simulink model "faults"  (R2023b)
settings: Solver=VariableStepAuto  StartTime=0.0  StopTime=10.0  RelTol=1e-3
libraries: spsSeriesRLCBranchLib x4, spsThreePhaseBreakerLib x1, spsThreePhaseFaultLib x1, spsUniversalBridgeLib x1
settings Model: Creator=edemk  LastModifiedBy=edemk

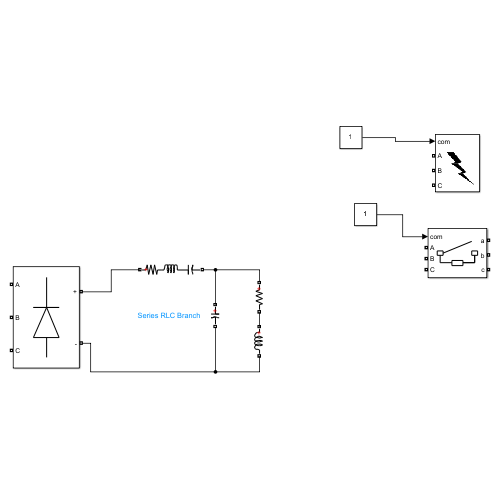
[thumbnail: Simulink's stored preview of the top-level diagram]
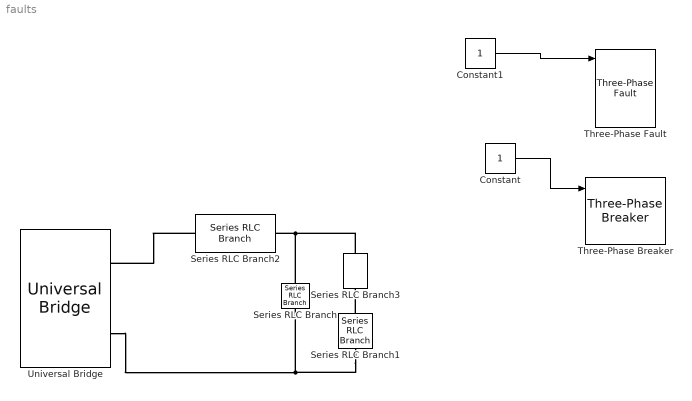
== system faults ==
  Constant : Constant
  Constant1 : Constant
  Series RLC Branch : spsSeriesRLCBranchLib/Series RLC Branch  LConnTagsString=__new0  RConnTagsString=__new0  BranchType=C  Resistance=1  Inductance=1e-3  SetiL0=off  InitialCurrent=0  Capacitance=1e-6  Setx0=off  InitialVoltage=0  Measurements=None
  Series RLC Branch1 : spsSeriesRLCBranchLib/Series RLC Branch  LConnTagsString=__new0  RConnTagsString=__new0  BranchType=L  Resistance=1  Inductance=1e-3  SetiL0=off  InitialCurrent=0  Capacitance=1e-6  Setx0=off  InitialVoltage=0  Measurements=None
  Series RLC Branch2 : spsSeriesRLCBranchLib/Series RLC Branch  LConnTagsString=__new0  RConnTagsString=__new0  BranchType=RLC  Resistance=1  Inductance=1e-3  SetiL0=off  InitialCurrent=0  Capacitance=1e-6  Setx0=off  InitialVoltage=0  Measurements=None
  Series RLC Branch3 : spsSeriesRLCBranchLib/Series RLC Branch  LConnTagsString=__new0  RConnTagsString=__new0  BranchType=R  Resistance=1  Inductance=1e-3  SetiL0=off  InitialCurrent=0  Capacitance=1e-6  Setx0=off  InitialVoltage=0  Measurements=None
  Three-Phase Breaker : spsThreePhaseBreakerLib/Three-Phase Breaker  InitialState=open  SwitchA=on  SwitchB=on  SwitchC=on  SwitchTimes="[1/60  5/60]"  External=on  BreakerResistance=0.1  SnubberResistance=0.1  SnubberCapacitance=inf  Measurements=Breaker voltages and currents
  Three-Phase Fault : spsThreePhaseFaultLib/Three-Phase Fault  InitialStates=1  FaultA=on  FaultB=on  FaultC=on  GroundFault=off  SwitchTimes="[1/60  5/60]"  External=on  SwitchStatus=NaN  FaultResistance=0.0001  GroundResistance=0.01  SnubberResistance=0.0001  SnubberCapacitance=inf  Measurements=Fault voltages and currents
  Universal Bridge : spsUniversalBridgeLib/Universal Bridge  Arms=3  SnubberResistance=1e5  SnubberCapacitance=inf  Device=Diodes  Ron=1e-3  Lon=0  ForwardVoltages="[  0  0  ]"  ForwardVoltage=0  GTOparameters=[ 10e-6 , 20e-6 ]  IGBTparameters=[ 1e-6 , 2e-6 ]  Measurements=None  Measurements_2=None  converterType=Rectifier
  wires:
  Constant/1 -> Three-Phase Breaker/1
  Constant1/1 -> Three-Phase Fault/1
  connections:
  Series RLC Branch1/LConn1 -- Series RLC Branch3/RConn1
  Series RLC Branch3/LConn1 -- Series RLC Branch/LConn1 -- Series RLC Branch2/RConn1
  Series RLC Branch1/RConn1 -- Series RLC Branch/RConn1 -- Universal Bridge/RConn2
  Series RLC Branch2/LConn1 -- Universal Bridge/RConn1
